simulink model "SIM004_DIMENSIONAL"  (R2019a)
settings: Solver=FixedStepAuto  StartTime=0.0  StopTime=50  FixedStep=0.0001  RelTol=1e-3
values from neighbouring files (symbols this model uses):
  A = 4    [SIM002.m]    (also in SIM004_DIMENSIONAL_PARAMS.m = 12)
  C_x0 = 1.1856    [SIM002.m]    (also in SIM004_DIMENSIONAL_PARAMS.m)
  C_y1 = 0.3842    [SIM002.m]    (also in SIM004_DIMENSIONAL_PARAMS.m)
  D = 0.08    [SIM001.m]    (also in SIM002.m; SIM004_DIMENSIONAL_PARAMS.m)
  epsilon = 0.05    [SIM002.m]    (also in SIM004_DIMENSIONAL_PARAMS.m = 0.7)
  kt = 0.032    [SIM001.m]    (also in SIM004_DIMENSIONAL_PARAMS.m = 0.1)
  omega_n = sqrt(k/M)    [SIM001.m]    (also in SIM002.m; SIM004_DIMENSIONAL_PARAMS.m)
  omega_s = 2*pi*fs    [SIM002.m]    (also in SIM004_DIMENSIONAL_PARAMS.m)
  P = (m_star + Cm)*2*pi^3*St^2    (= 8.46208055933)    [SIM002.m]    (also in SIM004_DIMENSIONAL_PARAMS.m = rho_w*D*L*U^2/(2*M))
  r2 = 0.01    [SIM001.m]    (also in SIM004_DIMENSIONAL_PARAMS.m)
  U = Vr*(fn*D)    [SIM001.m]    (also in SIM002.m = Vn*fn*D; SIM004_DIMENSIONAL_PARAMS.m = Vn*fn*D)
  zeta = b/(2*omega_n*M)    [SIM002.m]    (also in SIM004_DIMENSIONAL_PARAMS.m = c/(2*omega_n*M))
libraries: powerlib x5, powerlib_meascontrol x1
settings Model: Creator=dinet  LastModifiedBy=dinet

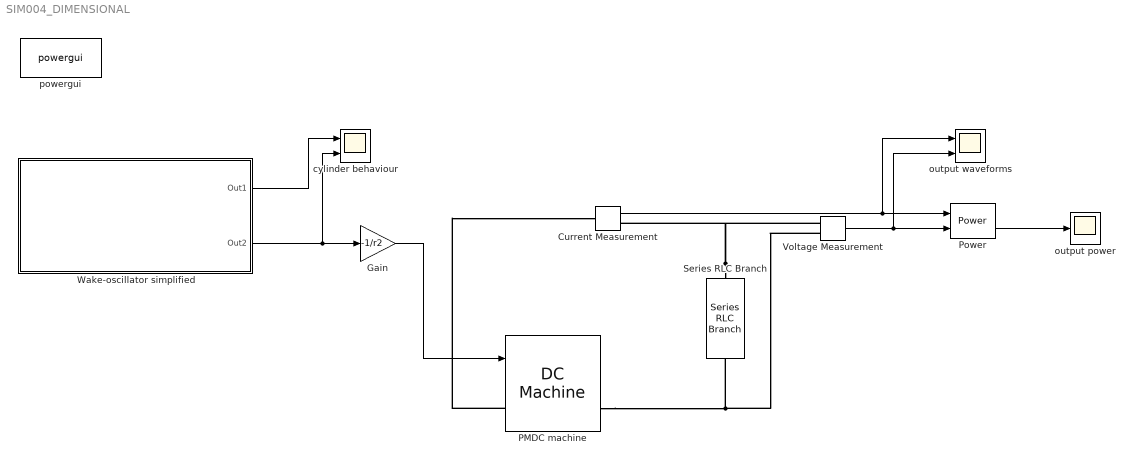
== system SIM004_DIMENSIONAL ==
  Current Measurement : powerlib/Measurements/Current Measurement  PhasorSimulation=off  OutputType=Complex  PSBequivalent=0
      settings: SourceProductName=Simscape Electrical
  Gain : Gain  Gain=-1/r2
  "PMDC machine " : powerlib/Machines/DC Machine  PresetModel=No  MechanicalLoad=Speed w  FieldType=Permanent magnet  ShowDetailedParameters=on  MeasurementBus=off  RLa="[ 0.6  0.012]"  RLf="[ 240  120]"  Laf=1.8  MachineConstant=Torque constant (N.m/A)  Ke=0.003  Kt=kt  J=1  Bm=0  Tf=0  w0=1  Ifinit=1  TsPowergui=0  TsBlock=-1
      settings: SourceProductName=Simscape Electrical
  Power : powerlib_meascontrol/Measurements/Power  Freq=1  Vinit=[0, 0]  Iinit=[0, 0]  Ts=0
      settings: SourceProductName=Simscape Electrical
  Series RLC Branch : powerlib/Elements/Series RLC Branch  LConnTagsString=__new0  RConnTagsString=__new0  BranchType=R  Resistance=100  Inductance=0  SetiL0=off  InitialCurrent=0  Capacitance=0  Setx0=off  InitialVoltage=0  Measurements=None
      settings: SourceProductName=Simscape Electrical
  Voltage Measurement : powerlib/Measurements/Voltage Measurement  PhasorSimulation=off  OutputType=Complex  PSBequivalent=0
      settings: SourceProductName=Simscape Electrical
  Wake-oscillator simplified : Subsystem
  cylinder behaviour : Scope  NumInputPorts=2
  output power : Scope
  output waveforms : Scope  NumInputPorts=2
  powergui : powerlib/powergui  Priority=1  SimulationMode=Continuous  SampleTime=50e-6  frequency=60  Iterations=50  frequencyindice=0  Pbase=100e6  ErrMax=1e-4  UnitsV=kV  UnitsW=MW  buscounter=0  FunctionMessages=off  echomessages=off  EnableUseOfTLC=off  CurrentSourceSwitches=off  DisableSnubberDevices=off  DisableRonSwitches=off  DisableVfSwitches=off  DisplayEquations=off  AutomaticDiscreteSolvers=off  SolverType=Tustin/Backward Euler (TBE)  Interpol=off  ExternalGateDelay=off  methode=off  Ts=100  x0status=blocks  SPID=on  SwTol=0  HookPort=off  NonlinearTolerance=0  nMaxIteration=15  ContinueOnMaxIteration=off  RestoreLinks=warning  ResistiveCurrentMeasurement=off  Frange=[0:2:500]  Ylog=off  Xlog=on  ShowGrid=off  save=off  variable=ZData  structure=0  ZoomFFT=off  StartTime=0.0  cycles=1  DisplayStyle=1  fundamental=60  FreqAxis=off  MaxFrequency=1000  frequencyindicesteady=1  RmsSteady=1  display=off
      settings: SourceProductName=Simscape Electrical
  wires:
  Voltage Measurement/1 -> output waveforms/2, Power/1
  Power/1 -> output power/1
  Current Measurement/1 -> output waveforms/1, Power/2
  Gain/1 -> "PMDC machine "/1
  Wake-oscillator simplified/1(Out1) -> cylinder behaviour/1
  Wake-oscillator simplified/2(Out2) -> Gain/1, cylinder behaviour/2
  connections:
  Series RLC Branch/LConn1 -- Voltage Measurement/LConn1 -- Current Measurement/RConn1
  "PMDC machine "/RConn1 -- Voltage Measurement/LConn2 -- Series RLC Branch/RConn1
  "PMDC machine "/LConn1 -- Current Measurement/LConn1

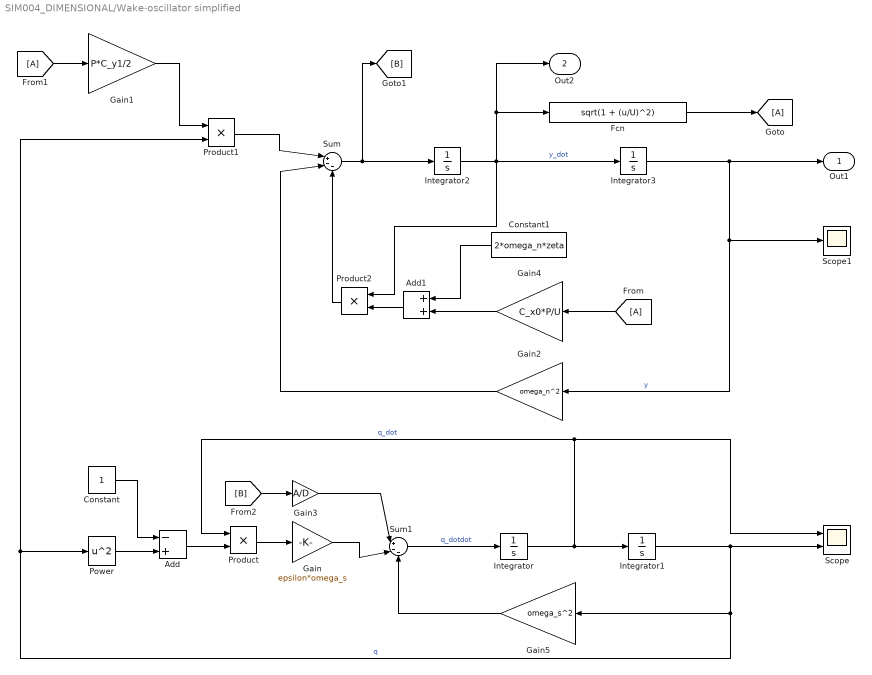
== system SIM004_DIMENSIONAL/Wake-oscillator simplified ==
  Add : Sum  Inputs=-+
  Add1 : Sum
  Constant : Constant
  Constant1 : Constant  Value=2*omega_n*zeta
  Fcn : Fcn  Expr=sqrt(1 + (u/U)^2)
  Gain : Gain  Gain=epsilon*omega_s
  Gain1 : Gain  Gain=P*C_y1/2
  Gain2 : Gain  Gain=omega_n^2
  Gain3 : Gain  Gain=A/D
  Gain4 : Gain  Gain=C_x0*P/U
  Gain5 : Gain  Gain=omega_s^2
  Integrator : Integrator
  Integrator1 : Integrator  InitialCondition=0.001
  Integrator2 : Integrator
  Integrator3 : Integrator
  Power : Math  Operator=square  SaturateOnIntegerOverflow=on
  Product : Product
  Product1 : Product
  Product2 : Product
  Scope : Scope  NumInputPorts=2
  Scope1 : Scope
  Sum : Sum  Inputs=|+--
  Sum1 : Sum  Inputs=|+--
  Out1 : Outport
  Out2 : Outport  Port=2
  wires:
  Integrator3/1 -> Scope1/1, Gain2/1, Out1/1  "y"
  Gain1/1 -> Product1/1
  Integrator/1 -> Integrator1/1, Product/1, Scope/1  "q_dot"
  Gain5/1 -> Sum1/3
  Sum1/1 -> Integrator/1  "q_dotdot"
  Gain4/1 -> Add1/2
  [B] -> Gain3/1
  Integrator1/1 -> Scope/2, Power/1, Product1/2, Gain5/1  "q"
  Gain3/1 -> Sum1/1
  Sum/1 -> Integrator2/1, [B]
  Integrator2/1 -> Fcn/1, Out2/1, Integrator3/1, Product2/1  "y_dot"
  Add/1 -> Product/2
  Add1/1 -> Product2/2
  Product/1 -> Gain/1
  Power/1 -> Add/2
  Product1/1 -> Sum/1
  Gain/1 -> Sum1/2
  [A] -> Gain4/1
  Fcn/1 -> [A]
  [A] -> Gain1/1
  Constant1/1 -> Add1/1
  Constant/1 -> Add/1
  Product2/1 -> Sum/3
  Gain2/1 -> Sum/2
